simulink subsystem "linear"  (R2023a)
settings: Solver=VariableStepAuto  StartTime=0.0  StopTime=10.0  RelTol=1e-3
undefined symbols (not defined in the file): Ard, Brd, Crd, x_ic
settings Model: Creator=pinki  LastModifiedBy=pinki

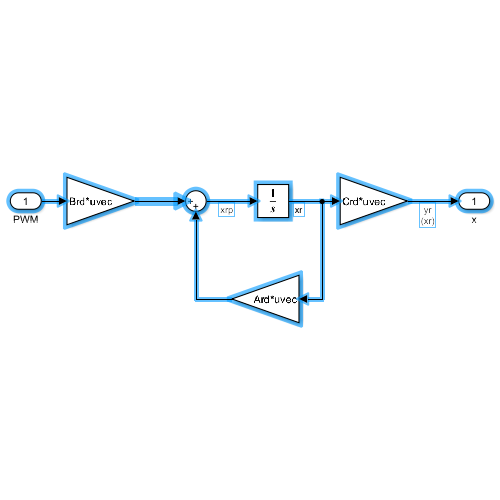
[thumbnail: Simulink's stored preview of the top-level diagram]
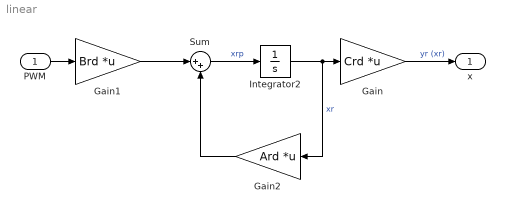
== system linear ==
  PWM : Inport
  Gain : Gain  Gain=Crd  Multiplication=Matrix(K*u) (u vector)
  Gain1 : Gain  Gain=Brd  Multiplication=Matrix(K*u) (u vector)
  Gain2 : Gain  Gain=Ard  Multiplication=Matrix(K*u) (u vector)
  Integrator2 : Integrator  InitialCondition=x_ic
  Sum : Sum  Inputs=|++
  x : Outport
  wires:
  PWM/1 -> Gain1/1
  Sum/1 -> Integrator2/1  "xrp"
  Gain/1 -> x/1  "yr (xr)"
  Integrator2/1 -> Gain2/1, Gain/1  "xr"
  Gain2/1 -> Sum/2
  Gain1/1 -> Sum/1
